simulink model "test_model"  (R2026a)
settings: Solver=FixedStepAuto  StopTime=inf  FixedStep=0.002
model workspace (MAT data in the model file):
  SL_ROS_VariableLengthArrays_MaxSizes.CommonInfo.ArrayTruncateAction = 'EmitWarning'
  SL_ROS_VariableLengthArrays_MaxSizes.MsgTypeMap = containers.Map
  SL_ROS_VariableLengthArrays_MaxSizes.MsgTypeMap.serialization.keys = {'sensor_msgs/Image', 'sensor_msgs/LaserScan'}
  SL_ROS_VariableLengthArrays_MaxSizes.MsgTypeMap.serialization.values{1}(1).PropertyName = 'data'
  SL_ROS_VariableLengthArrays_MaxSizes.MsgTypeMap.serialization.values{1}(1).DataType = 'uint8'
  SL_ROS_VariableLengthArrays_MaxSizes.MsgTypeMap.serialization.values{1}(1).MaxLength = 921600
  SL_ROS_VariableLengthArrays_MaxSizes.MsgTypeMap.serialization.values{1}(2).PropertyName = 'encoding'
  SL_ROS_VariableLengthArrays_MaxSizes.MsgTypeMap.serialization.values{1}(2).DataType = 'uint8'
  SL_ROS_VariableLengthArrays_MaxSizes.MsgTypeMap.serialization.values{1}(2).MaxLength = 128
  SL_ROS_VariableLengthArrays_MaxSizes.MsgTypeMap.serialization.values{2}(1).PropertyName = 'intensities'
  SL_ROS_VariableLengthArrays_MaxSizes.MsgTypeMap.serialization.values{2}(1).DataType = 'single'
  SL_ROS_VariableLengthArrays_MaxSizes.MsgTypeMap.serialization.values{2}(1).MaxLength = 640
  SL_ROS_VariableLengthArrays_MaxSizes.MsgTypeMap.serialization.values{2}(2).PropertyName = 'ranges'
  SL_ROS_VariableLengthArrays_MaxSizes.MsgTypeMap.serialization.values{2}(2).DataType = 'single'
  SL_ROS_VariableLengthArrays_MaxSizes.MsgTypeMap.serialization.values{2}(2).MaxLength = 640
  SL_ROS_VariableLengthArrays_MaxSizes.MsgTypeMap.serialization.uniformity = 0
  SL_ROS_VariableLengthArrays_MaxSizes.MsgTypeMap.serialization.keyType = 'char'
  SL_ROS_VariableLengthArrays_MaxSizes.MsgTypeMap.serialization.valueType = 'any'
undefined symbols (not defined in the file): angular, gray, linear
libraries: ros2lib x6
settings Model: Creator=Erin  LastModifiedBy=Erin

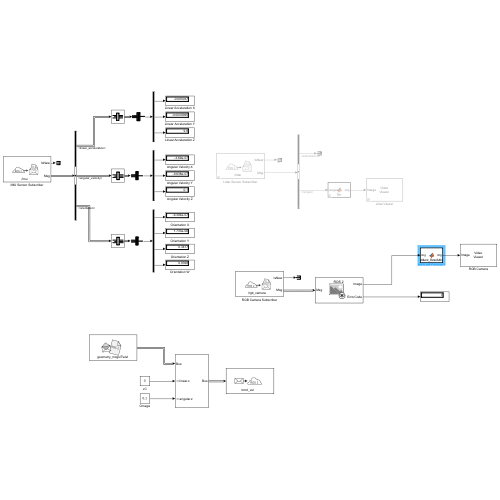
[thumbnail: Simulink's stored preview of the top-level diagram]
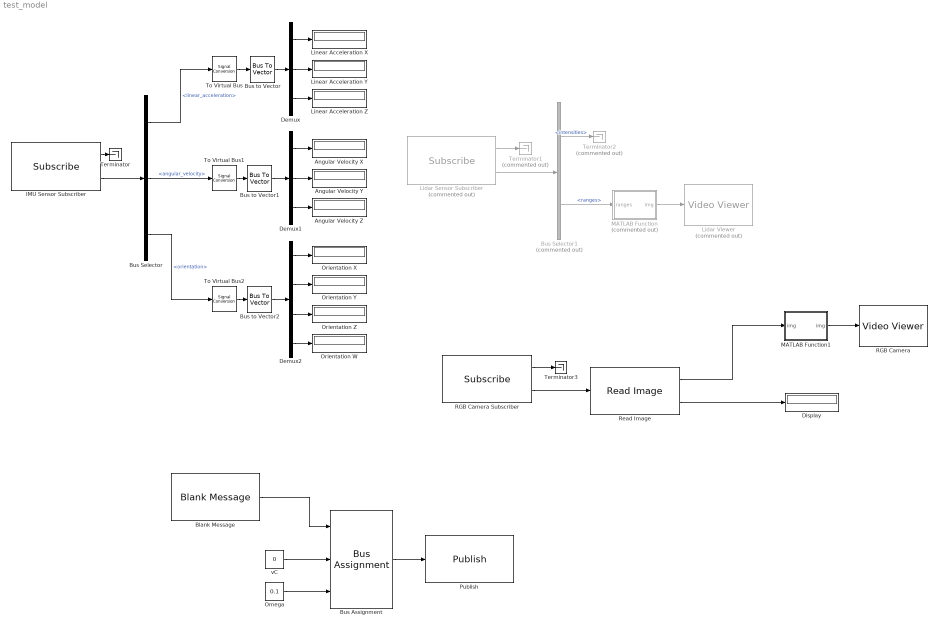
== system test_model ==
  Angular Velocity X : Display
  Angular Velocity Y : Display
  Angular Velocity Z : Display
  Blank Message : ros2lib/Blank Message  messageClass=Message  entityType=geometry_msgs/Twist  messageType=geometry_msgs/Twist  SampleTime=inf
  Bus Assignment : BusAssignment  AssignedSignals=linear.x,angular.z
  Bus Selector : BusSelector  OutputSignals=linear_acceleration,angular_velocity,orientation
  Bus Selector1 : BusSelector  Commented=on  OutputSignals=intensities,ranges
  Bus to Vector : BusToVector
  Bus to Vector1 : BusToVector
  Bus to Vector2 : BusToVector
  Demux : Demux  Outputs=3
  Demux1 : Demux  Outputs=3
  Demux2 : Demux
  Display : Display
  IMU Sensor Subscriber : ros2lib/Subscribe  topicSource=Select from ROS network  topic=/imu  messageType=sensor_msgs/Imu  sampleTime=-1  QOSHistory=Keep last  QOSDepth=10  QOSReliability=Reliable  QOSDurability=Volatile  QOSDeadline=Inf  QOSLifespan=Inf  QOSLiveliness=Automatic  QOSLeaseDuration=Inf  QOSAvoidROSNamespaceConventions=off
  Lidar Sensor Subscriber : ros2lib/Subscribe  Commented=on  topicSource=Select from ROS network  topic=/lidar  messageType=sensor_msgs/LaserScan  sampleTime=-1  QOSHistory=Keep last  QOSDepth=10  QOSReliability=Reliable  QOSDurability=Volatile  QOSDeadline=Inf  QOSLifespan=Inf  QOSLiveliness=Automatic  QOSLeaseDuration=Inf  QOSAvoidROSNamespaceConventions=off
  Lidar Viewer : VideoViewer  Commented=on  colormapValue=gray(256)  FigPos=[-713 975 418 304]
  Linear Acceleration X : Display
  Linear Acceleration Y : Display
  Linear Acceleration Z : Display
  MATLAB Function : MATLAB Function  Commented=on  TreatAsAtomicUnit=on
  MATLAB Function1 : MATLAB Function  TreatAsAtomicUnit=on
  Omega : Constant  Value=0.1
  Orientation W : Display
  Orientation X : Display
  Orientation Y : Display
  Orientation Z : Display
  Publish : ros2lib/Publish  topicSource=Specify your own  topic=/cmd_vel  messageType=geometry_msgs/Twist  QOSHistory=Keep last  QOSDepth=10  QOSReliability=Reliable  QOSDurability=Volatile  QOSDeadline=Inf  QOSLifespan=Inf  QOSLiveliness=Automatic  QOSLeaseDuration=Inf  QOSAvoidROSNamespaceConventions=off
  RGB Camera : VideoViewer  colormapValue=gray(256)  FigPos=[-721 470 418 304]
  RGB Camera Subscriber : ros2lib/Subscribe  topicSource=Select from ROS network  topic=/rgb_camera  messageType=sensor_msgs/Image  sampleTime=-1  QOSHistory=Keep last  QOSDepth=10  QOSReliability=Reliable  QOSDurability=Volatile  QOSDeadline=Inf  QOSLifespan=Inf  QOSLiveliness=Automatic  QOSLeaseDuration=Inf  QOSAvoidROSNamespaceConventions=off
  Read Image : ros2lib/Read Image  MaximumImageSize=[480, 640]  ImageEncoding=rgb8  ShowAlphaOutput=off  ShowErrorCodeOutput=on  VariableSizeOutputs=off
  Terminator : Terminator
  Terminator1 : Terminator  Commented=on
  Terminator2 : Terminator  Commented=on
  Terminator3 : Terminator
  To Virtual Bus : SignalConversion  ConversionOutput=Virtual bus  OverrideOpt=off
  To Virtual Bus1 : SignalConversion  ConversionOutput=Virtual bus  OverrideOpt=off
  To Virtual Bus2 : SignalConversion  ConversionOutput=Virtual bus  OverrideOpt=off
  vC : Constant  Value=0
  wires:
  IMU Sensor Subscriber/1 -> Terminator/1
  IMU Sensor Subscriber/2 -> Bus Selector/1
  Demux/3 -> Linear Acceleration Z/1
  Demux/2 -> Linear Acceleration Y/1
  Demux/1 -> Linear Acceleration X/1
  Demux1/3 -> Angular Velocity Z/1
  Demux1/2 -> Angular Velocity Y/1
  Demux1/1 -> Angular Velocity X/1
  Bus Selector/2 -> To Virtual Bus1/1  "<angular_velocity>"
  Demux2/2 -> Orientation Y/1
  Demux2/1 -> Orientation X/1
  Demux2/4 -> Orientation W/1
  Demux2/3 -> Orientation Z/1
  Omega/1 -> Bus Assignment/3
  Bus Assignment/1 -> Publish/1
  vC/1 -> Bus Assignment/2
  Blank Message/1 -> Bus Assignment/1
  Lidar Sensor Subscriber/1 -> Terminator1/1
  Lidar Sensor Subscriber/2 -> Bus Selector1/1
  Bus Selector/1 -> To Virtual Bus/1  "<linear_acceleration>"
  Bus to Vector/1 -> Demux/1
  Bus to Vector1/1 -> Demux1/1
  Bus to Vector2/1 -> Demux2/1
  To Virtual Bus/1 -> Bus to Vector/1
  To Virtual Bus1/1 -> Bus to Vector1/1
  To Virtual Bus2/1 -> Bus to Vector2/1
  Bus Selector/3 -> To Virtual Bus2/1  "<orientation>"
  Bus Selector1/1 -> Terminator2/1  "<intensities>"
  Bus Selector1/2 -> MATLAB Function/1(ranges)  "<ranges>"
  MATLAB Function/1(img) -> Lidar Viewer/1
  RGB Camera Subscriber/1 -> Terminator3/1
  RGB Camera Subscriber/2 -> Read Image/1
  Read Image/2 -> Display/1
  MATLAB Function1/1(img) -> RGB Camera/1
  Read Image/1 -> MATLAB Function1/1("img ")

== matlab function test_model/MATLAB Function ==
  data: ranges input; img output
function img = fcn(ranges)

img = ranges'/10;

== matlab function test_model/MATLAB Function1 ==
  data: img input; img output
function img = Reduce_Resolution(img)

[m,n] = size(img);

img = img(1:10:m, 1:10:n);
